simulink model "Connection"  (R2022a)
settings: Solver=VariableStepAuto  StartTime=0.0  StopTime=60  RelTol=1e-3
libraries: dspsrcs4 x7, whdledac x2, whdlutilities x1
settings Model: Creator=Zeyan Wu  LastModifiedBy=Zeyan

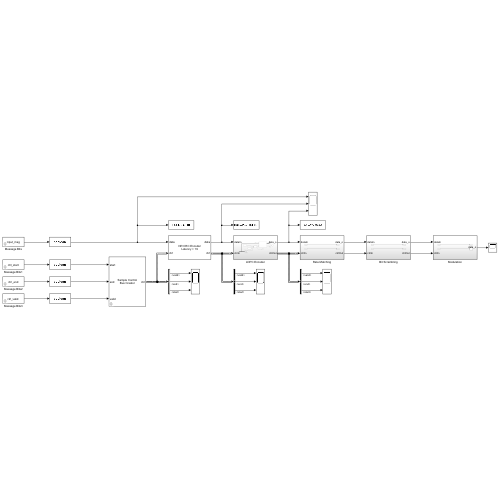
[thumbnail: Simulink's stored preview of the top-level diagram]
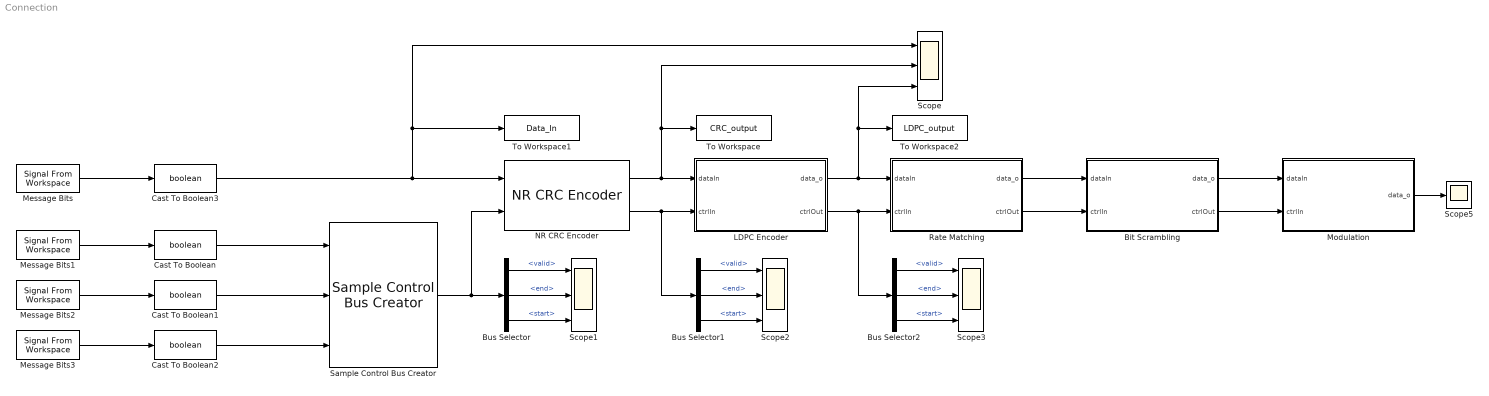
== system Connection ==
  Bit Scrambling : Subsystem
  Bus Selector : BusSelector  OutputSignals=valid,end,start
  Bus Selector1 : BusSelector  OutputSignals=valid,end,start
  Bus Selector2 : BusSelector  OutputSignals=valid,end,start
  Cast To Boolean{,1..3} (4 alike) : DataTypeConversion  OutDataTypeStr=boolean  SaturateOnIntegerOverflow=off  RndMeth=Floor
  LDPC Encoder : Subsystem
  Message Bits : dspsrcs4/Signal From Workspace  X=input_msg  Ts=1  nsamps=1  OutputAfterFinalValue=Setting to zero  ignoreOrWarnInputAndFrameLengths=off  OutputFrames=on
  Message Bits1 : dspsrcs4/Signal From Workspace  X=ctrl_start  Ts=1  nsamps=1  OutputAfterFinalValue=Setting to zero  ignoreOrWarnInputAndFrameLengths=off  OutputFrames=on
  Message Bits2 : dspsrcs4/Signal From Workspace  X=ctrl_end  Ts=1  nsamps=1  OutputAfterFinalValue=Setting to zero  ignoreOrWarnInputAndFrameLengths=off  OutputFrames=on
  Message Bits3 : dspsrcs4/Signal From Workspace  X=ctrl_valid  Ts=1  nsamps=1  OutputAfterFinalValue=Setting to zero  ignoreOrWarnInputAndFrameLengths=off  OutputFrames=on
  Modulation : Subsystem
  NR CRC Encoder : whdledac/NR CRC Encoder  CRCType=CRC16  EnableCRCMaskPort=off  SimulateUsing=Code generation
      settings: SourceProductBaseCode=LH
  Rate Matching : Subsystem
  Sample Control Bus Creator : whdlutilities/Sample Control Bus Creator
      settings: SourceProductBaseCode=LH
  Scope{,1..3} (4 alike) : Scope  NumInputPorts=3
  Scope5 : Scope
  To Workspace : ToWorkspace  VariableName=CRC_output  SampleTime=1
      settings: Save2DSignal=2-D array (concatenate along first dimension)
  To Workspace1 : ToWorkspace  VariableName=Data_In  SampleTime=1
      settings: Save2DSignal=2-D array (concatenate along first dimension)
  To Workspace2 : ToWorkspace  VariableName=LDPC_output  SampleTime=1
      settings: Save2DSignal=2-D array (concatenate along first dimension)
  wires:
  Message Bits2/1 -> Cast To Boolean1/1
  Message Bits1/1 -> Cast To Boolean/1
  Message Bits3/1 -> Cast To Boolean2/1
  Sample Control Bus Creator/1 -> Bus Selector/1, NR CRC Encoder/2
  Cast To Boolean/1 -> Sample Control Bus Creator/1
  Cast To Boolean1/1 -> Sample Control Bus Creator/2
  Cast To Boolean2/1 -> Sample Control Bus Creator/3
  Bus Selector/1 -> Scope1/1  "<valid>"
  Bus Selector/3 -> Scope1/3  "<start>"
  NR CRC Encoder/1 -> LDPC Encoder/1(dataIn), Scope/2, To Workspace/1
  Bus Selector/2 -> Scope1/2  "<end>"
  Message Bits/1 -> Cast To Boolean3/1
  Cast To Boolean3/1 -> Scope/1, To Workspace1/1, NR CRC Encoder/1
  Bus Selector1/2 -> Scope2/2  "<end>"
  NR CRC Encoder/2 -> Bus Selector1/1, LDPC Encoder/2(ctrlIn)
  Bus Selector1/3 -> Scope2/3  "<start>"
  Bus Selector1/1 -> Scope2/1  "<valid>"
  Bus Selector2/2 -> Scope3/2  "<end>"
  Bus Selector2/3 -> Scope3/3  "<start>"
  Bus Selector2/1 -> Scope3/1  "<valid>"
  LDPC Encoder/1(data_o) -> Scope/3, To Workspace2/1, Rate Matching/1(dataIn)
  LDPC Encoder/2(ctrlOut) -> Rate Matching/2(ctrlIn), Bus Selector2/1
  Rate Matching/1(data_o) -> Bit Scrambling/1(dataIn)
  Rate Matching/2(ctrlOut) -> Bit Scrambling/2(ctrlIn)
  Bit Scrambling/1(data_o) -> Modulation/1(dataIn)
  Bit Scrambling/2(ctrlOut) -> Modulation/2(ctrlIn)
  Modulation/1(data_o) -> Scope5/1

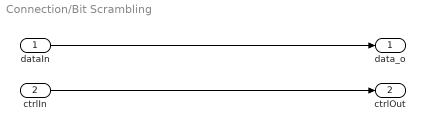
== system Connection/Bit Scrambling ==
  dataIn : Inport
  ctrlIn : Inport  Port=2
  data_o : Outport
  ctrlOut : Outport  Port=2
  wires:
  dataIn/1 -> data_o/1
  ctrlIn/1 -> ctrlOut/1

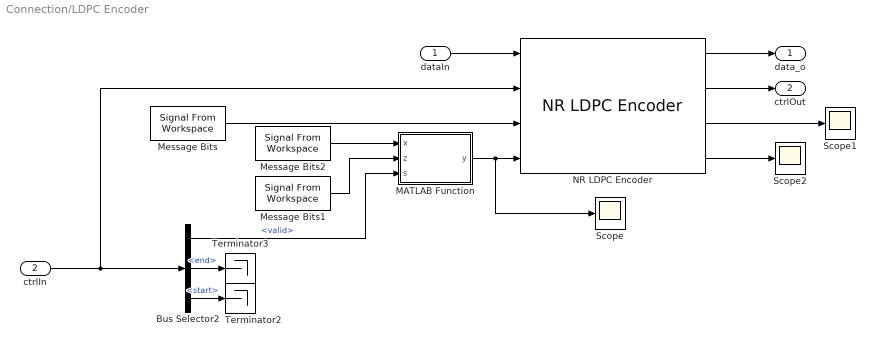
== system Connection/LDPC Encoder ==
  dataIn : Inport
  ctrlIn : Inport  Port=2
  Bus Selector2 : BusSelector  OutputSignals=valid,end,start
  MATLAB Function : MATLAB Function  TreatAsAtomicUnit=on
  Message Bits : dspsrcs4/Signal From Workspace  X=BGN  Ts=1  nsamps=1  OutputAfterFinalValue=Holding final value  ignoreOrWarnInputAndFrameLengths=off  OutputFrames=on
  Message Bits1 : dspsrcs4/Signal From Workspace  X=liftingSize  Ts=1  nsamps=1  OutputAfterFinalValue=Holding final value  ignoreOrWarnInputAndFrameLengths=off  OutputFrames=on
  Message Bits2 : dspsrcs4/Signal From Workspace  X=liftingSize_zero  Ts=1  nsamps=1  OutputAfterFinalValue=Holding final value  ignoreOrWarnInputAndFrameLengths=off  OutputFrames=on
  NR LDPC Encoder : whdledac/NR LDPC Encoder
      settings: SourceProductBaseCode=LH
  Scope : Scope
  Scope1 : Scope
  Scope2 : Scope
  Terminator2 : Terminator
  Terminator3 : Terminator
  data_o : Outport
  ctrlOut : Outport  Port=2
  wires:
  NR LDPC Encoder/2 -> ctrlOut/1
  dataIn/1 -> NR LDPC Encoder/1
  NR LDPC Encoder/1 -> data_o/1
  NR LDPC Encoder/3 -> Scope1/1
  NR LDPC Encoder/4 -> Scope2/1
  Message Bits/1 -> NR LDPC Encoder/3
  ctrlIn/1 -> NR LDPC Encoder/2, Bus Selector2/1
  Bus Selector2/3 -> Terminator2/1  "<start>"
  Bus Selector2/2 -> Terminator3/1  "<end>"
  Bus Selector2/1 -> MATLAB Function/3(s)  "<valid>"
  MATLAB Function/1(y) -> Scope/1, NR LDPC Encoder/4
  Message Bits2/1 -> MATLAB Function/1(x)
  Message Bits1/1 -> MATLAB Function/2(z)

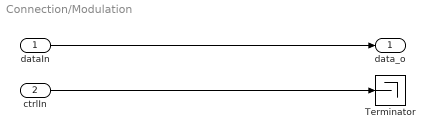
== system Connection/Modulation ==
  dataIn : Inport
  ctrlIn : Inport  Port=2
  Terminator : Terminator
  data_o : Outport
  wires:
  dataIn/1 -> data_o/1
  ctrlIn/1 -> Terminator/1

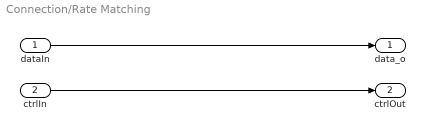
== system Connection/Rate Matching ==
  dataIn : Inport
  ctrlIn : Inport  Port=2
  data_o : Outport
  ctrlOut : Outport  Port=2
  wires:
  dataIn/1 -> data_o/1
  ctrlIn/1 -> ctrlOut/1

== matlab function Connection/LDPC Encoder/MATLAB Function ==
  data: x input; y output; z input; s input
function y = selector(x, z, s)
    if(s == false)
        y = x;
    else
        y = z;
    end
end
